simulink model "MPC_Validation_2_ISNM"  (R2020a)
settings: Solver=FixedStepAuto  StartTime=0.0  StopTime=tsim  FixedStep=baseRate  RelTol=1e-3  EnableMultiTasking=on
values from neighbouring files (symbols this model uses):
  Ad = -C(7:12,4:9)    [theFastMPCSolver3.m]
  ALGORITHM = 5    [Run_Initializer.m]    (also in main.m = 7)
  baseRate = 0.05    [Run_Initializer.m]
  con0 = [n*N, 2*N, N, N, N]    [Run_Initializer.m]    (also in main.m)
  drop_states_ARM = [ pi/2, pi/2, 0]    [Run_Initializer.m]
  drop_states_BLACK = rand([1,3])/10+init_states_BLACK    [Run_Initializer.m]
  drop_states_BLUE = rand([1,3])/10+init_states_BLUE    [Run_Initializer.m]
  drop_states_RED = rand([1,3])/10+init_states_RED    [Run_Initializer.m]
  F_Black_X_nominal = 0.2196    [Run_Initializer.m]
  F_Black_Y_nominal = 0.2825    [Run_Initializer.m]
  F_Blue_X_nominal = 0.2196    [Run_Initializer.m]
  F_Blue_Y_nominal = 0.2825    [Run_Initializer.m]
  F_red_X_nominal = 0.2196    [Run_Initializer.m]
  F_red_Y_nominal = 0.2825    [Run_Initializer.m]
  F_thrusters_BLACK = [F_Black_X_nominal; F_Black_X_nominal;                             F_Black_Y_nominal; F_Black_Y_nominal; F_Black_X_nominal;                              F_Black_X_nominal; F_Black_Y_nominal; F_Black_Y_nominal]    [Run_Initializer.m]
  F_thrusters_BLUE = [F_Blue_X_nominal; F_Blue_X_nominal;                             F_Blue_Y_nominal; F_Blue_Y_nominal; F_Blue_X_nominal;                              F_Blue_X_nominal; F_Blue_Y_nominal; F_Blue_Y_nominal]    [Run_Initializer.m]
  F_thrusters_RED = [F_red_X_nominal; F_red_X_nominal;                             F_red_Y_nominal; F_red_Y_nominal; F_red_X_nominal;                              F_red_X_nominal; F_red_Y_nominal; F_red_Y_nominal]    [Run_Initializer.m]
  gamma = r - (excess + shrink + bracketwidth)    [theChaserSpacecraft.m]    (also in theTargetSpacecraft.m)
  Gamma1 = 0.0025    [Run_Initializer.m]
  Gamma2 = 100    [Run_Initializer.m]
  Gamma3 = 10    [Run_Initializer.m]
  Gamma4 = 0.001    [Run_Initializer.m]
  Gamma5 = 100    [Run_Initializer.m]
  Gamma6 = 0.001    [Run_Initializer.m]
  init_states_BLACK = [ct;thetat0].'    [Run_Initializer.m]
  init_states_BLUE = [pobj1;0].'    [Run_Initializer.m]
  init_states_RED = xi(1:3).'    [Run_Initializer.m]
  Kd_elarm = 0.05    [Run_Initializer.m]
  Kd_sharm = 0.05    [Run_Initializer.m]
  Kd_tb = 0.4    [Run_Initializer.m]
  Kd_tblue = 0.4    [Run_Initializer.m]
  Kd_tr = 0.4    [Run_Initializer.m]
  Kd_wrarm = 0.005    [Run_Initializer.m]
  Kd_xb = 8    [Run_Initializer.m]
  Kd_xblue = 8    [Run_Initializer.m]
  Kd_xr = 8    [Run_Initializer.m]
  Kd_yb = 8    [Run_Initializer.m]
  Kd_yblue = 8    [Run_Initializer.m]
  Kd_yr = 8    [Run_Initializer.m]
  Kp = [0.08 0 0 ... (first row only)    [Run_Initializer.m]
  Kp_elarm = 0.08    [Run_Initializer.m]
  Kp_sharm = 0.15    [Run_Initializer.m]
  Kp_tb = 0.1    [Run_Initializer.m]
  Kp_tblue = 0.1    [Run_Initializer.m]
  Kp_tr = 0.1    [Run_Initializer.m]
  Kp_wrarm = 0.007    [Run_Initializer.m]
  Kp_xb = 2    [Run_Initializer.m]
  Kp_xblue = 2    [Run_Initializer.m]
  Kp_xr = 2    [Run_Initializer.m]
  Kp_yb = 2    [Run_Initializer.m]
  Kp_yblue = 2    [Run_Initializer.m]
  Kp_yr = 2    [Run_Initializer.m]
  Kv = [0.05 0 0 ... (first row only)    [Run_Initializer.m]
  maxiterations = 10    [Run_Initializer.m]    (also in main.m)
  N = 15    [Run_Initializer.m]    (also in main.m; theFastMPCSolver2.m = length(z)/9; theFastMPCSolver3.m = length(z)/9)
  n = size(b,1)    [theFastMPCSolver3.m]
  noise_variance_BLACK = 0    [Run_Initializer.m]
  noise_variance_BLUE = 0    [Run_Initializer.m]
  noise_variance_RED = 0    [Run_Initializer.m]
  Phase0_End = Phase0_Duration    (= 5)    [Run_Initializer.m]
  Phase1_End = Phase0_Duration + Phase1_Duration    (= 10)    [Run_Initializer.m]
  Phase2_End = Phase0_Duration + Phase1_Duration +                                   Phase2_Duration    (= 36)    [Run_Initializer.m]
  Phase3_End = Phase0_Duration + Phase1_Duration +                                   Phase2_Duration + Phase3_Duration    (= 166)    [Run_Initializer.m]
  Phase3_SubPhase1_End = Phase2_End + Phase3_SubPhase1_Duration    (= 40)    [Run_Initializer.m]
  Phase3_SubPhase2_End = Phase2_End + Phase3_SubPhase1_Duration +                                   Phase3_SubPhase2_Duration    (= 42)    [Run_Initializer.m]
  Phase3_SubPhase3_End = Phase2_End + Phase3_SubPhase1_Duration +                                   Phase3_SubPhase2_Duration +                                  Phase3_SubPhase3_Duration    (= 44)    [Run_Initializer.m]
  Phase3_SubPhase4_End = Phase2_End + Phase3_SubPhase1_Duration +                                   Phase3_SubPhase2_Duration +                                  Phase3_SubPhase3_Duration +                                  Phase3_SubPhase4_Duration    [Run_Initializer.m]
  Phase4_End = Phase0_Duration + Phase1_Duration +                                   Phase2_Duration + Phase3_Duration +                                   Phase4_Duration    (= 186)    [Run_Initializer.m]
  Phase5_End = Phase0_Duration + Phase1_Duration +                                   Phase2_Duration + Phase3_Duration +                                   Phase4_Duration + Phase5_Duration    (= 191)    [Run_Initializer.m]
  serverRate = 0.1    [Run_Initializer.m]
  Td = 2    [Run_Initializer.m]    (also in main.m)
  thetat_dot = 0 * d2r    (= 0)    [Run_Initializer.m]    (also in main.m = -2.0 * d2r)
  thruster_dist2CG_BLACK = [83.42;-52.58;55.94;-60.05;54.08;-53.92;77.06;-55.94]    [Run_Initializer.m]
  thruster_dist2CG_BLUE = [73.54;-64.46;81.39;-60.11;64.46;-65.94;54.61;-74.39]    [Run_Initializer.m]
  thruster_dist2CG_RED = [49.92;-78.08;70.46;-63.54;81.08;-50.42;57.44;-75.96]    [Run_Initializer.m]
  tol = 0.00015    [Run_Initializer.m]    (also in main.m)
  Tz_lim_elarm = .1    (= 0.1)    [Run_Initializer.m]
  Tz_lim_sharm = .1    (= 0.1)    [Run_Initializer.m]
  Tz_lim_wrarm = .1    (= 0.1)    [Run_Initializer.m]
  vobj1 = [0.00;0.00]    [Run_Initializer.m]    (also in main.m)
  vtar = [0.0;0.0]    [Run_Initializer.m]    (also in main.m = [-0.008;0.008])
undefined symbols (not defined in the file or in its folder): cdockdeltax, cdockoa, Cmat, DiscIntNeverNeededParam, ecoa, Fmat, H, KOZ_actual, model_param, pdockoa, pdockr, platformSelection, rcone, rdock, simMode, Sj, taumax, thetah, Umat, umax, WhoAmI
libraries: dspstat3 x23, dspsigops x15, embdlinuxlib x10, raspberrypiBasiclib x10, simulink x8, MainLibrary x7, mspfiltlib x3, dsparch4 x3, dspswit3 x2, sensehatlib x1
(part 14 of 14)

== matlab function MPC_Validation_2_ISNM/Triggered Subsystem/MPC ==
  data: CONTROL output; xi input; Td parameter; N parameter; pdockr parameter; rdock parameter; thetah parameter; KOZ_actual parameter; Sj parameter; rcone parameter; Ad parameter; con0 parameter; Cmat parameter; Umat parameter; Fmat parameter; H parameter; gamma parameter; tol parameter; x0 output; rhold output; x0 input; rhold input; ALGORITHM parameter; umax parameter; taumax parameter; n parameter; ct input; pobj1 input; vtar input; vobj1 input; thetat0 input; thetat_dot input; pdockoa parameter; ecoa parameter; cdockoa parameter; maxiterations parameter; CPUTIME output; cdockdeltax parameter
function [CONTROL, x0, rhold, CPUTIME] = MPC(xi,Td, N, pdockr, rdock, thetah, KOZ_actual, Sj, rcone, Ad, con0, Cmat, Umat, Fmat, H, gamma, tol, x0, rhold, ALGORITHM, umax, taumax, n, ct, pobj1, vtar, vobj1, thetat0, thetat_dot, pdockoa, ecoa, cdockoa, maxiterations, cdockdeltax)
    % COPY-PASTED FROM LOOP IN MAIN
    d2r = pi/180;
    
    N = 15;
    maxiterations = 10;
    
    % The moving target and obstacle positions for the current sampling instant, k
    [pobj1hz, ptar] = theMovingObstacleHorizonParameters(Td,N,ct,pobj1,vtar,vobj1);
    
    % The rotating target parameters for the current sampling instant, k
    [thetat,m1,m2,nc1,nc2,pdock,xt,cdock] = theRotatingTargetHorizonParameters(Td,N,ptar,vtar,pdockr,rhold,rdock,cdockoa,pdockoa,ecoa,thetat_dot,thetah,thetat0,cdockdeltax);
    
%     % Compare the angles in the same [0,2pi] range
% %     xi(6:9:end) = wrapTo2Pi(xi(6:9:end));
%     positiveInput = (xi(3) > 0);
%     lambda = mod(xi(3), 2*pi);
%     lambda((lambda == 0) & positiveInput) = 2*pi;
%     xi(3) = lambda;
% 
%     positiveInput = (x0(6:9:9*N) > 0);
%     lambda = mod(x0(6:9:9*N), 2*pi);
%     lambda((lambda == 0) & positiveInput) = 2*pi;
%     x0(6:9:9*N) = lambda;
%     
% %     xt(6:9:end) = wrapTo2Pi(xt(6:9:end));
%     positiveInput = (xt(3:6:6*N) > 0);
%     lambda = mod(xt(3:6:6*N), 2*pi);
%     lambda((lambda == 0) & positiveInput) = 2*pi;
%     xt(3:6:6*N) = lambda;
%     %thetat = wrapToPi(thetat);
    
    % Reshape the xt variable for use in theObjectiveFunction, ignore the
    % current state and reform into [03 xt(2) 03 xt(2) 03 ... 03 xt(N+1)]
    xt9 = zeros(9,N);
    xt9(4:9,:) = xt(:,2:N+1);
    xt9 = reshape(xt9, [9*N,1]);
    
    % The reference trajectory of the chaser over the horizon of instant k
    pxref = theReferenceTrajectory(x0,N); % 2xN

    % The points ro on the KOZ boundaries of the obstacles over the horizon
    ro_1 = theObstacleLinearizer(pxref,pobj1hz(:,2:N+1),KOZ_actual);
    ro_t = theObstacleLinearizer(pxref,ptar(:,2:N+1),rhold);
    
    % Reshape pdock for use in the linearized matrix constraints
    pdock9 = zeros(9,N);
    pdock9(4:5,:) = pdock(:,2:N+1);
    pdock9 = reshape(pdock9, [9*N,1]);

    % Make the ro_X and robj9 vectors for obstacle constraints
    ro_1_9 = zeros(9,N);
    ro_1_9(4:5,:) = ro_1;
    ro_1_9 = reshape(ro_1_9,9*N,1);

    ro_t_9 = zeros(9,N);
    ro_t_9(4:5,:) = ro_t;
    ro_t_9 = reshape(ro_t_9,9*N,1);

    robj1_9 = zeros(9,N);
    robj1_9(4:5,:) = pobj1hz(:,2:N+1);
    robj1_9 = reshape(robj1_9,9*N,1);

    rtar_9 = zeros(9,N);
    rtar_9(4:5,:) = ptar(:,2:N+1);
    rtar_9 = reshape(rtar_9,9*N,1);

    % Make the matrix for obstacle constraints
    S1 = Sj;
    St = [1/(rhold*rhold), 0; 0, 1/(rhold*rhold)];

    E1 = (ro_1 - pobj1hz(:,2:N+1)).' * S1;
    Et = (ro_t - ptar(:,2:N+1)).' * St;

    D1 = zeros(N,(9*N));
    Dt = zeros(N,(9*N));
    for row = 1:N
        D1(row,4+(row-1)*9:5+(row-1)*9) = E1(row,:);
        Dt(row,4+(row-1)*9:5+(row-1)*9) = Et(row,:);
    end  
    
    % Define the b vector for Cx = b dynamics constraint
    bvec = zeros(6*N,1);
    bvec(1:6) = Ad*xi;
    
    % Define arrays for the hyperplane normal arrays to be used for the entry cone constraints
    nc1m = zeros(N,9*N);
    nc2m = zeros(N,9*N);
        
    % Determine if the entry cone constraints should be on
    if ((xi(1:2) - cdock(1:2,1)).' * (xi(1:2) - cdock(1:2,1)) < rcone*rcone) % if chaser is within rcone range
        
        temp1 = -nc1(2,:) * x0(4:5) + nc1(2,:) * pdock9(4:5);
        temp2 = nc2(2,:) * x0(4:5) - nc2(2,:) * pdock9(4:5);
        
              
        if temp1 <= 0 && temp2 <= 0 % only turn ec constraints on if it won't cause infeasibilities at the next step
            
        
            withEntryCone = 1; % turn on
            con = [n*N, 2*N, N, N, N, N, N];

            % Create Nx2N matrix of the entry cone normal to each hyperplane
            % Should be in the form
            % ncm = [ 0_1x3 n1_1x2 0_1x4 0_1x3  0_1x2 0_1x4  ... 0_1x3 0_1x2 0_1x4
            %         0_1x3  0_1x2 0_1x4 0_1x3 n2_1x2 0_1x4  ... 0_1x3 0_1x2 0_1x4
            %                           ...
            %         0_1x3  0_1x2 0_1x4 0_1x3  0_1x2 0_1x4  ... 0_1x3 nN+1_1x2 0_1x4
            for i=1:N
                nc1m(i,4+(i-1)*9:5+(i-1)*9) = nc1(i+1,:);
                nc2m(i,4+(i-1)*9:5+(i-1)*9) = nc2(i+1,:);
            end
        else
            
            withEntryCone = 0; % turn off
            con = con0;

            % FOR PLOTTING PURPOSES
            m1 = NaN;
            m2 = NaN;
        end
                
    else
        withEntryCone = 0; % turn off
        con = con0;
        
        % FOR PLOTTING PURPOSES
        m1 = NaN;
        m2 = NaN;
    end
    

    
%     if ALGORITHM == 5     
        % Constraint Matrix
%         if ~withEntryCone
%             Wmat = [-2*D1;-2*Dt];
%         else
%             Wmat = [-2*D1;-2*Dt;-nc1m;nc2m];
%         end
%     % THIS NEEDS TO BE CLEANED UP
%     elseif ALGORITHM == 6 || ALGORITHM == 7
        if withEntryCone
            Wmat = zeros(10*N,9*N);
            hvec = zeros(10*N,1);
        else
            Wmat = zeros(8*N,9*N);
            hvec = zeros(8*N,1);
        end

        for index = 0:N-1
            blockc = 9*index;
            if withEntryCone
                blockr = 10*index;
                Wmat(9+blockr,:) = -nc1m(index+1,:);
                Wmat(10+blockr,:) = nc2m(index+1,:);
            else
                blockr = 8*index;
            end
            Wmat(1+blockr:3+blockr,1+blockc:3+blockc) = eye(3);
            Wmat(4+blockr:6+blockr,1+blockc:3+blockc) = -eye(3);
            Wmat(7+blockr,:) = -2*D1(index+1,:);
            Wmat(8+blockr,:) = -2*Dt(index+1,:);
        end

        f_D1 = -ones(N,1) - D1*(ro_1_9 + robj1_9);
        f_Dt = -ones(N,1) - Dt*(ro_t_9 + rtar_9);   
        if withEntryCone % if entry cone constraints turned on
            f_ec1 = -nc1m * pdock9;
            f_ec2 = nc2m * pdock9;
        else
            f_ec1 = NaN;
            f_ec2 = NaN;
        end

        for index = 0:N-1
            if withEntryCone % if entry cone constraints turned on
                blockr = 10*index;
                hvec(9+blockr) = f_ec1(index+1);
                hvec(10+blockr) = f_ec2(index+1);
            else
                blockr = 8*index;
            end

            hvec(1+blockr:3+blockr) = [umax;umax;taumax];
            hvec(4+blockr:6+blockr) = [umax;umax;taumax];
            hvec(7+blockr) = f_D1(index+1);
            hvec(8+blockr) = f_Dt(index+1);
        end
% 
%     end
    
    % Constraint upper and lower limits
%     if ALGORITHM == 5
%         [cl,cu,bineqvec] = theConstraintLimits4(Umat,Fmat,Wmat,con0,con,...
%             D1,Dt,ro_1_9,ro_t_9,robj1_9,rtar_9,nc1m,...
%             nc2m,pdock9);
%     end
    
    

%     
%     % Ensure a feasible start
%     if ALGORITHM == 6 || ALGORITHM == 7
%         if any((hvec - Wmat*x0) <= 0)
% %             disp('Started with infeasible solution (outside).');
%             infeas0 = find((hvec - Wmat*x0) <= 0);
%             disp(infeas0)
% 
%             % Find a new feasible z-val for the violated constraint(s)
%             for ind = infeas0.'
%                 if size(con) == size(con0) % no ec constraints yet
%                     ind_startrange = 7 + 8*idivide(ind,int16(8+1));
%                     ind_endrange = ind_startrange + 1;
%                 else
%                     ind_startrange = 7 + 10*idivide(ind,int16(10+1));
%                     ind_endrange = ind_startrange + 3;
%                 end
% %                 disp(ind_startrange)
% %                 disp(ind_endrange)
%                     
%                 z_infeas_ind = find(Wmat(ind,:)); % optimization variable(s) to vary
%     %             disp('z(infeas)=')
%     %             disp(z_infeas_ind)
% 
%                 newind = z_infeas_ind - 9;
%                 
%                 search_range = 1;
%                 search_stepnum = 1001;
%                 
%                 while (1)
%                     if newind < 0
% %                         disp("Sampling...")
% 
%                         % make a grid of search points
%                         try_x = linspace(x0(z_infeas_ind(1))-search_range,x0(z_infeas_ind(1))+search_range,search_stepnum);
%                         try_y = linspace(x0(z_infeas_ind(2))-search_range,x0(z_infeas_ind(2))+search_range,search_stepnum);
%                         [xx,yy] = meshgrid(try_x,try_y);
% 
%                         % calcuate the constraint at each grid point
% %                         temp = zeros(search_stepnum,search_stepnum);
%                         temp2 = zeros(search_stepnum*search_stepnum,3);
%                         for i1=1:search_stepnum
%                             for i2 = 1:search_stepnum
%                                 temp = hvec(ind_startrange:ind_endrange) - Wmat(ind_startrange:ind_endrange,z_infeas_ind)*[xx(i1,i2);yy(i1,i2)];
% 
%                                 % take note of grid points that satisfy the constraint
%                                 if ~any(temp <= 0)
%                                     temp2((i1-1)*search_stepnum+i2,1) = min(temp);
%                                     temp2((i1-1)*search_stepnum+i2,2) = i1;
%                                     temp2((i1-1)*search_stepnum+i2,3) = i2;
%                                 end
%                             end
%                         end
% 
%                         % get rid of data that does not satisfy the constraints
%                         temp2( ~any(temp2,2), : ) = [];  %rows
%                         
%                         if isempty(temp2)
%                             search_range = 3;
%                             search_stepnum = search_stepnum * 2;
%                             continue
%                         end
% 
%                         % choose one of the grid points that satisfy the constraint
%                         % currently finds the first minimum value... could be further improved
%                         ind_of_min = find(temp2(:,1) == min(temp2(:,1)));
%                         ind_chosen = ind_of_min(1);
% 
%                         % update the x0 with the new grid point
%                         [i1i2_chosen] = temp2(ind_chosen,[2,3]);
%                         i1_chosen = i1i2_chosen(1);
%                         i2_chosen = i1i2_chosen(2);
%                         x0(z_infeas_ind) = [xx(i1_chosen,i2_chosen);yy(i1_chosen,i2_chosen)];                     
%                         
%                     else
%                         x0(z_infeas_ind) = x0(newind); % re-tracing previous sol'n
%                     end
% 
%                     if (hvec(ind)- Wmat(ind,:)*x0) <= 0
%                         if newind < 0
%                             continue
%                         else
%                             newind = newind - 9;
%                         end
%                     else
% %                         disp("Resolved.")
%                         break
%                         
%                     end
%                 end
%             end
%         end
%        
%     end
%     
%     
%     
%     % Setup Options
%     if ALGORITHM == 5
%         options = optimoptions('quadprog','Algorithm','active-set','MaxIterations',10);
%     elseif ALGORITHM == 6 || ALGORITHM == 7
        nu = zeros(6*N,1);
%     end
%     
%     % Solve!
%     if ALGORITHM == 5
%         tic
%         [x,fval] = quadprog(H,-H.'*xt9,Wmat,bineqvec,Cmat,bvec,cl,cu,x0,options);
%         CPUTIME = toc;
%     elseif ALGORITHM == 6
%         disp('----------------------------------------------')
%         disp(string(count))
%         
        tic
        [x,nu] = theFastMPCSolver2(x0,nu,xt9,H,Cmat,bvec,Wmat,hvec,1e-9,0.01,0.95,maxiterations);
        CPUTIME = toc;
%     elseif ALGORITHM == 7
%         disp('----------------------------------------------')
%         disp(string(count))
%         tic
%         [x,nu] = theFastMPCSolver3(x0,nu,xt9,H,Cmat,bvec,Wmat,hvec,1e-9,0.01,0.95,maxiterations);
%         CPUTIME = toc;
%     end
   

    % Save data
%     sol(end+1:end+9) = x(1:9);
%     soliter(1:n,count) = xi;
%     soliter(n+1:n+9*N,count) = x;
%     solpobj(count,1) = pobj1hz(1,1); 
%     solpobj(count,2) = pobj1hz(2,1);
%     solpobj(count,3) = pobj2hz(1,1);
%     solpobj(count,4) = pobj2hz(2,1);
%     solptar(count,1) = ptar(1,1);
%     solptar(count,2) = ptar(2,1);
%     solm1(count,1) = m1(1);
%     solm2(count,1) = m2(1);
%     solthetat(count,1) = thetat(1);
%     solpdock(count,1:2) = pdock(:,1);
%     if ALGORITHM == 0
%         solJ(end+1) = theObjectiveFunction0(x,N,xt,P,Q,R);
%     elseif ALGORITHM > 0
%         solJ(end+1) = theObjectiveFunction123(x,xt9,H);
%     end
%     count = count + 1;

    CONTROL = x(1:3);
    
    % Determine if the chaser is docked using the 'current' positions of
    % the chaser and docking condition; done using only position
    if (xi(1:2) - cdock(1:2,1)).' * (xi(1:2) - cdock(1:2,1)) < tol
        isdocked = 1;
    end
    
    % Set the next guess as the solution from the previous iteration
    xi = x(4:9); % the next 'current' state of the chaser spacecraft
    % x0 = [x(10:end);0;0;0;Ad*x0(4+9*(N-2):9+9*(N-2)) + Bd*x0(1+9*(N-1):3+9*(N-1))];
    x0 = [x(10:end);0;0;0;x(4+9*(N-1):9+9*(N-1))];
    
    % Update rhold if:
    %  - the position of the chaser matches the holding position, within tolerance
    %  - the attitude of the chaser matches the docking condition, within tolerance
    %  - the holding radius is larger than its minimum allowable size, rdock
    if abs((xi(1:2) - xt(1:2,1)).' * (xi(1:2) - xt(1:2,1))) < 0.5 % if position error is below tolerance
        if abs(xi(3) - cdock(3,1)) < 10*d2r % if attitude error is below tolerance
            if rhold > rdock
                rhold = rhold * gamma; % decrease the holding radius
                if rhold < rdock
                    rhold = rdock; % set to the minimum holding radius, rdock
                end
            end
        end
    end
    
    % Set the next 'current' target and obstacle positions
%     ct = ptar(:,2);
%     pobj1 = pobj1hz(:,2); 
%     pobj2 = pobj2hz(:,2);
        
    % Set the new target theta value for the next iteration
%     thetat0 = thetat(2);
    
end

== matlab function MPC_Validation_2_ISNM/From Force//Torque to PWM Signal/Change BLUE Behavior/Calculate Thruster ON//OFF/MATLAB Function1 ==
  data: H output; thruster_dist2CG_BLUE parameter; F_thrusters_BLUE parameter
function H = MakeH(thruster_dist2CG_BLUE,F_thrusters_BLUE)

Vec1 = [ -1
         -1
          0 
          0
          1
          1
          0
          0 ];
      
Vec2 = [  0
          0
          1
          1
          0
          0
         -1
         -1 ];
     
Vec3 = thruster_dist2CG_BLUE./1000;

Mat1 = [Vec1, Vec2, Vec3]';

Mat2 = diag((F_thrusters_BLUE./2));

H    = Mat1*Mat2;

end
